simulink model "LKAS_AutoSave_DF_20220408_1006_SW62"  (R2018b)
settings: Solver=FixedStepDiscrete  StartTime=0.0  StopTime=10.0  FixedStep=0.01  RelTol=1e-3
undefined symbols (not defined in the file): LKA_CarWidth, LKA_SampleTime, LKA_StrRatio_C, LKA_Veh2CamL_C, LKA_Veh2CamW_C, LKA_WhlBaseL_C, LL_CompHdAg_C, LL_CompSWA_C, LL_CrvtPrvwT_C, LL_DesDvt_C, LL_DvtComp_C, LL_DvtPrvwT_C, LL_DvtSpdDet_vDvtSpdMin_C, LL_HandsOff_ExitTime, LL_HandsOff_TextTime, LL_HandsOff_WarnTime, LL_HdAgExT_C, LL_HdAgPrvwT_C, LL_LAccMax_C, LL_LAccRMax_C, LL_LDW_EarliestWarnLine_C, LL_LDW_LatestWarnLine_C, LL_LDWS_SUPPRESS_HEADING, LL_LFClb_TFC_FfCtlRatio_C, LL_LFClb_TFC_KdBalance_C, LL_LFClb_TFC_KdMaxSWA_C, LL_LFClb_TFC_KdV1_C, LL_LFClb_TFC_KdV2_C, LL_LFClb_TFC_KdVehSpdLwr_C, LL_LFClb_TFC_KdVehSpdUpr_C, LL_LFClb_TFC_Ki_C, LL_LFClb_TFC_KiMaxSWA_C, LL_LFClb_TFC_Kp_C, LL_LFClb_TFC_KpKlat_C, LL_LFClb_TFC_KpV1_C, LL_LFClb_TFC_KpV2_C, LL_LFClb_TFC_KpVehSpdLwr_C, LL_LFClb_TFC_KpVehSpdUpr_C, LL_LFClb_TFC_PrvwT_C, LL_LKA_EarliestWarnLine_C, LL_LKA_LatestWarnLine_C, LL_LKAExPrcs_ExitC0Dvt, LL_LKAExPrcs_ExitC0Swt, LL_LKAExPrcs_tiExitDelayTime3, LL_LKAExPrcs_tiExitTime1, LL_LKAExPrcs_tiExitTime2, LL_LKAExPrcs_tiExitTime3, LL_LKAS_OUT_OF_CONTROL_LAT_VEL, LL_LKAS_OUT_OF_CONTROL_TTLC, LL_LKASWASyn_M0, LL_LKASWASyn_M1, LL_LKASWASyn_M2, LL_LKASWASyn_M3D, LL_LKASWASyn_M3K_DT, LL_LKASWASyn_M3K_MSD, LL_LKASWASyn_M4K, LL_LKASWASyn_SWAaddMax, LL_LKASWASyn_T2, LL_LKASWASyn_tiTrqSwaRtTime, LL_LKASWASyn_tiTrqSwaTime ... (+47)
libraries: simulink x234, canmsglib x6, dspstat3 x3, simulink_extras x1
(part 5 of 16)

== system LKAS_AutoSave_DF_20220408_1006_SW62/LKAS/LL/Fault_Diagnostic/FuncFaultStatus_Unpack ==
  note: ob_ADIA_SpareDataCheck
  FuncFaultStatus : Inport
  Bus Creator : BusCreator  Inputs=16
  Extract Bits : simulink/Logic and Bit Operations/Extract Bits  bitsToExtract=Range of bits  numBits=8  bitIdxRange=0  outScalingMode=Treat bit field as an integer
      settings: SourceProductName=Simulink
  Extract Bits1 : simulink/Logic and Bit Operations/Extract Bits  bitsToExtract=Range of bits  numBits=8  bitIdxRange=1  outScalingMode=Treat bit field as an integer
      settings: SourceProductName=Simulink
  Extract Bits10 : simulink/Logic and Bit Operations/Extract Bits  bitsToExtract=Range of bits  numBits=8  bitIdxRange=10  outScalingMode=Treat bit field as an integer
      settings: SourceProductName=Simulink
  Extract Bits11 : simulink/Logic and Bit Operations/Extract Bits  bitsToExtract=Range of bits  numBits=8  bitIdxRange=11  outScalingMode=Treat bit field as an integer
      settings: SourceProductName=Simulink
  Extract Bits12 : simulink/Logic and Bit Operations/Extract Bits  bitsToExtract=Range of bits  numBits=8  bitIdxRange=12  outScalingMode=Treat bit field as an integer
      settings: SourceProductName=Simulink
  Extract Bits13 : simulink/Logic and Bit Operations/Extract Bits  bitsToExtract=Range of bits  numBits=8  bitIdxRange=13  outScalingMode=Treat bit field as an integer
      settings: SourceProductName=Simulink
  Extract Bits14 : simulink/Logic and Bit Operations/Extract Bits  bitsToExtract=Range of bits  numBits=8  bitIdxRange=14  outScalingMode=Treat bit field as an integer
      settings: SourceProductName=Simulink
  Extract Bits15 : simulink/Logic and Bit Operations/Extract Bits  bitsToExtract=Range of bits  numBits=8  bitIdxRange=15  outScalingMode=Treat bit field as an integer
      settings: SourceProductName=Simulink
  Extract Bits2 : simulink/Logic and Bit Operations/Extract Bits  bitsToExtract=Range of bits  numBits=8  bitIdxRange=2  outScalingMode=Treat bit field as an integer
      settings: SourceProductName=Simulink
  Extract Bits3 : simulink/Logic and Bit Operations/Extract Bits  bitsToExtract=Range of bits  numBits=8  bitIdxRange=3  outScalingMode=Treat bit field as an integer
      settings: SourceProductName=Simulink
  Extract Bits4 : simulink/Logic and Bit Operations/Extract Bits  bitsToExtract=Range of bits  numBits=8  bitIdxRange=4  outScalingMode=Treat bit field as an integer
      settings: SourceProductName=Simulink
  Extract Bits5 : simulink/Logic and Bit Operations/Extract Bits  bitsToExtract=Range of bits  numBits=8  bitIdxRange=5  outScalingMode=Treat bit field as an integer
      settings: SourceProductName=Simulink
  Extract Bits6 : simulink/Logic and Bit Operations/Extract Bits  bitsToExtract=Range of bits  numBits=8  bitIdxRange=6  outScalingMode=Treat bit field as an integer
      settings: SourceProductName=Simulink
  Extract Bits7 : simulink/Logic and Bit Operations/Extract Bits  bitsToExtract=Range of bits  numBits=8  bitIdxRange=7  outScalingMode=Treat bit field as an integer
      settings: SourceProductName=Simulink
  Extract Bits8 : simulink/Logic and Bit Operations/Extract Bits  bitsToExtract=Range of bits  numBits=8  bitIdxRange=8  outScalingMode=Treat bit field as an integer
      settings: SourceProductName=Simulink
  Extract Bits9 : simulink/Logic and Bit Operations/Extract Bits  bitsToExtract=Range of bits  numBits=8  bitIdxRange=9  outScalingMode=Treat bit field as an integer
      settings: SourceProductName=Simulink
  bsFuncFaultStatus : Outport
  wires:
  Extract Bits9/1 -> Bus Creator/10
  Extract Bits6/1 -> Bus Creator/7
  Extract Bits7/1 -> Bus Creator/8
  Extract Bits3/1 -> Bus Creator/4
  Extract Bits4/1 -> Bus Creator/5
  Extract Bits8/1 -> Bus Creator/9  "ob_ADIA_SpareDataCheck"
  Extract Bits15/1 -> Bus Creator/16  "ob_DTC_AEB_Safety_Violation"
  Bus Creator/1 -> bsFuncFaultStatus/1  "bsFuncFaultStatus"
  Extract Bits/1 -> Bus Creator/1
  Extract Bits12/1 -> Bus Creator/13  "ob_DTC_ACC_Mixed_Mode_Conflict"
  Extract Bits11/1 -> Bus Creator/12  "ob_DTC_ACC_Accel_Decel_Safety_Violation"
  Extract Bits10/1 -> Bus Creator/11
  Extract Bits14/1 -> Bus Creator/15  "ob_DTC_ACC_HoldConfirm_Safety_Violation"
  Extract Bits5/1 -> Bus Creator/6
  Extract Bits13/1 -> Bus Creator/14  "ob_DTC_ACC_Displacement_Safety_Violation"
  Extract Bits1/1 -> Bus Creator/2
  Extract Bits2/1 -> Bus Creator/3
  FuncFaultStatus/1 -> Extract Bits15/1, Extract Bits14/1, Extract Bits13/1, Extract Bits12/1, Extract Bits11/1, Extract Bits10/1, Extract Bits9/1, Extract Bits8/1, Extract Bits7/1, Extract Bits6/1, Extract Bits5/1, Extract Bits4/1, Extract Bits3/1, Extract Bits2/1, Extract Bits1/1, Extract Bits/1

== system LKAS_AutoSave_DF_20220408_1006_SW62/LKAS/LL/Human Machine Interface (HMI)/Subsystem ==
  LDW_State : Inport
  LKA_State : Inport  Port=2
  bsEPSInfo : Inport  Port=3
  LKA_SampleTime : Inport  Port=4
  LL_HandsOff_TextTime : Inport  Port=5
  LL_HandsOff_WarnTime : Inport  Port=6
  LL_RlsDet_tiTrqChkT_DISABLE : Inport  Port=7
  LL_RlsDet_tiTrqChkT_EPS_DISABLE : Inport  Port=8
  Abs : Abs
  Bus Selector2 : BusSelector  OutputSignals=EPS_LKA_State,EPS_SW_Trq
  Compare{1..2,4,7} (4 alike) : simulink/Logic and Bit Operations/Compare To Constant  relop===  const=3  OutDataTypeStr=boolean
  Compare3 : simulink/Logic and Bit Operations/Compare To Constant  relop===  const=1  OutDataTypeStr=boolean
  Compare5 : simulink/Logic and Bit Operations/Compare To Constant  relop===  const=4  OutDataTypeStr=boolean
  Compare6 : simulink/Logic and Bit Operations/Compare To Constant  relop===  const=5  OutDataTypeStr=boolean
  Compare8 : simulink/Logic and Bit Operations/Compare To Constant  relop===  const=4  OutDataTypeStr=boolean
  Compare9 : simulink/Logic and Bit Operations/Compare To Constant  relop===  const=5  OutDataTypeStr=boolean
  Logical Operator1 : Logic  Operator=OR  AllPortsSameDT=off  OutDataTypeStr=boolean
  Logical Operator2 : Logic  Inputs=3  AllPortsSameDT=off  OutDataTypeStr=boolean
  Logical Operator3 : Logic  Operator=OR  Inputs=6  AllPortsSameDT=off  OutDataTypeStr=boolean
  Relational Operator : RelationalOperator  Operator=<=  OutDataTypeStr=boolean  RndMeth=Nearest
  Sum Condition1 : Subsystem  TreatAsAtomicUnit=on
  Sum Condition2 : Subsystem  TreatAsAtomicUnit=on
  Switch : Switch  Criteria=u2 > Threshold
  HandsOff2_Warn : Outport
  HandsOff1_Text : Outport  Port=2
  wires:
  LKA_SampleTime/1 -> [LKA_SampleTime]
  Bus Selector2/2 -> Abs/1  "<EPS_SW_Trq>"
  LL_HandsOff_WarnTime/1 -> Sum Condition2/2(Sum)
  LL_HandsOff_TextTime/1 -> Sum Condition1/2(Sum)
  [LKA_SampleTime] -> Sum Condition2/1(SampleTime), Sum Condition1/1(SampleTime)
  Logical Operator1/1 -> Logical Operator2/2
  Compare3/1 -> Logical Operator1/2
  Compare2/1 -> Logical Operator1/1
  Compare7/1 -> Logical Operator3/6
  Compare8/1 -> Logical Operator3/5
  Compare9/1 -> Logical Operator3/4
  LKA_State/1 -> Compare7/1, Compare8/1, Compare9/1
  Abs/1 -> Relational Operator/1
  Compare6/1 -> Logical Operator3/1
  Compare5/1 -> Logical Operator3/2
  Compare4/1 -> Logical Operator3/3
  LDW_State/1 -> Compare5/1, Compare6/1, Compare4/1
  Sum Condition2/1(Out) -> HandsOff2_Warn/1
  Relational Operator/1 -> Logical Operator2/3
  LL_RlsDet_tiTrqChkT_DISABLE/1 -> Switch/3
  Logical Operator3/1 -> Logical Operator2/1
  Logical Operator2/1 -> Sum Condition1/Enable, Sum Condition2/Enable
  Compare1/1 -> Switch/2
  Switch/1 -> Relational Operator/2
  bsEPSInfo/1 -> Bus Selector2/1
  LL_RlsDet_tiTrqChkT_EPS_DISABLE/1 -> Switch/1
  Bus Selector2/1 -> Compare1/1, Compare2/1, Compare3/1  "<EPS_LKA_State>"
  Sum Condition1/1(Out) -> HandsOff1_Text/1

== system LKAS_AutoSave_DF_20220408_1006_SW62/LKAS/LL/LL Inputs Mapping/bsBCMInfo ==
  bsBCMInfoIn : Inport
  Bus Creator1 : BusCreator  Inputs=3
  Bus Selector1 : BusSelector  OutputSignals=BCM_Double_Light,BCM_Left_Light,BCM_Right_Light,BCM_LeftTurn_Switch,BCM_RightTurn_Switch
  Compare To Constant : simulink/Logic and Bit Operations/Compare To Constant  relop===  const=1  OutDataTypeStr=boolean
  Compare To Constant1 : simulink/Logic and Bit Operations/Compare To Constant  relop===  const=1  OutDataTypeStr=boolean
  Logical Operator : Logic  Operator=OR  AllPortsSameDT=off  OutDataTypeStr=boolean
  Logical Operator1 : Logic  Operator=OR  AllPortsSameDT=off  OutDataTypeStr=boolean
  bsBCMInfoOut : Outport
  wires:
  Logical Operator1/1 -> Bus Creator1/3  "BCM_Right_Light"
  Logical Operator/1 -> Bus Creator1/2  "BCM_Left_Light"
  Compare To Constant1/1 -> Logical Operator1/2
  Compare To Constant/1 -> Logical Operator/2
  Bus Selector1/5 -> Compare To Constant1/1  "<BCM_RightTurn_Switch>"
  Bus Selector1/4 -> Compare To Constant/1  "<BCM_LeftTurn_Switch>"
  bsBCMInfoIn/1 -> Bus Selector1/1
  Bus Selector1/1 -> Bus Creator1/1  "<BCM_Double_Light>"
  Bus Creator1/1 -> bsBCMInfoOut/1
  Bus Selector1/2 -> Logical Operator/1  "<BCM_Left_Light>"
  Bus Selector1/3 -> Logical Operator1/1  "<BCM_Right_Light>"

== system LKAS_AutoSave_DF_20220408_1006_SW62/LKAS/LL/LL Inputs Mapping/bsEPSInfo ==
  bsEPSInfoIn : Inport
  Bus Creator4 : BusCreator  Inputs=11
  Bus Selector1 : BusSelector  OutputSignals=EPS_LKA_State,EPS_SW_Trq,EPS_Trq_State,SAS_Clb_State,SAS_Trim_State,SWS_Failure_Status,EPS_TrqLim_State,EPS_LKA_Current,EPS_SWHold_State,EPS_Driver_Override,EPS_ESA_State
  bsEPSInfoOut : Outport
  wires:
  Bus Selector1/11 -> Bus Creator4/11  "<EPS_ESA_State>"
  Bus Selector1/10 -> Bus Creator4/10  "<EPS_Driver_Override>"
  Bus Selector1/6 -> Bus Creator4/6  "<SWS_Failure_Status>"
  bsEPSInfoIn/1 -> Bus Selector1/1
  Bus Selector1/2 -> Bus Creator4/2  "<EPS_SW_Trq>"
  Bus Selector1/1 -> Bus Creator4/1  "<EPS_LKA_State>"
  Bus Creator4/1 -> bsEPSInfoOut/1
  Bus Selector1/3 -> Bus Creator4/3  "<EPS_Trq_State>"
  Bus Selector1/4 -> Bus Creator4/4  "<SAS_Clb_State>"
  Bus Selector1/5 -> Bus Creator4/5  "<SAS_Trim_State>"
  Bus Selector1/7 -> Bus Creator4/7  "<EPS_TrqLim_State>"
  Bus Selector1/8 -> Bus Creator4/8  "<EPS_LKA_Current>"
  Bus Selector1/9 -> Bus Creator4/9  "<EPS_SWHold_State>"

== system LKAS_AutoSave_DF_20220408_1006_SW62/LKAS/LL/LL Inputs Mapping/bsLaneInfo ==
  bsLLClb : Inport
  bsLaneInfoIn : Inport  Port=2
  Bus Creator : BusCreator  Inputs=5
  Bus Selector1 : BusSelector  OutputSignals=bsFusL0Info,bsFusR0Info,bsFusL1Info,bsFusR1Info,bsFusLrgInfo,bsFusRrgInfo,Fusion_AdditionalInf
  LaneSelect : Subsystem
  "LanesReconstruct " : Subsystem
  bsLaneInfoOut : Outport
  wires:
  LaneSelect/6(bsRrgInfo) -> "LanesReconstruct "/7(bsRrgInfo)
  LaneSelect/5(bsLrgInfo) -> "LanesReconstruct "/6(bsLrgInfo)
  Bus Selector1/6 -> LaneSelect/6(bsFusRrgInfo)  "<bsFusRrgInfo>"
  Bus Selector1/5 -> LaneSelect/5(bsFusLrgInfo)  "<bsFusLrgInfo>"
  bsLLClb/1 -> "LanesReconstruct "/1(bsLLClb)
  bsLaneInfoIn/1 -> Bus Selector1/1
  Bus Selector1/7 -> Bus Creator/5  "<Fusion_AdditionalInf>"
  "LanesReconstruct "/1(bsL0InfoR) -> Bus Creator/1  "bsL0Info"
  "LanesReconstruct "/2(bsR0InfoR) -> Bus Creator/2  "bsR0Info"
  "LanesReconstruct "/3(bsL1InfoR) -> Bus Creator/3  "bsL1Info"
  "LanesReconstruct "/4(bsR1InfoR) -> Bus Creator/4  "bsR1Info"
  LaneSelect/1(bsL0Info) -> "LanesReconstruct "/2(bsL0Info)
  LaneSelect/2(bsR0Info) -> "LanesReconstruct "/3(bsR0Info)
  LaneSelect/3(bsL1Info) -> "LanesReconstruct "/4(bsL1Info)
  LaneSelect/4(bsR1Info) -> "LanesReconstruct "/5(bsR1Info)
  Bus Selector1/1 -> LaneSelect/1(bsFusL0Info)  "<bsFusL0Info>"
  Bus Selector1/2 -> LaneSelect/2(bsFusR0Info)  "<bsFusR0Info>"
  Bus Selector1/3 -> LaneSelect/3(bsFusL1Info)  "<bsFusL1Info>"
  Bus Selector1/4 -> LaneSelect/4(bsFusR1Info)  "<bsFusR1Info>"
  Bus Creator/1 -> bsLaneInfoOut/1

== system LKAS_AutoSave_DF_20220408_1006_SW62/LKAS/LL/LL Inputs Mapping/bsMP5Info ==
  note: ELK_Mode
      | 0: off
      | 1: LDW
      | 2: ~
      | 3: ELK
  note: LKA_Mode
      | 0: off
      | 1: LDW
      | 2: LKA
  note: LKA_Mode
      | 0: LDW
      | 1: LKA
      | 2: ~
  note: LkaFcnConf
      | 0: OFF
      | 1: LDW-声音
      | 2: LDW-振动
      | 3: LDW-声音+振动
      | 4: LKA-声音
      | 5: LKA-振动
      | 6: LKA-声音+振动
      | 7: LDW-声音-ICA
      | 8: LDW-振动-ICA
      | 9: LDW-声音+振动-ICA
      | 10: LKA-声音-ICA
      | 11: LKA-振动-ICA
      | 12: LKA-声音+振动-ICA
  note: LDW_Warn_Mode
      | 0: 声音
      | 1: 振动
      | 2: 声音+振动
  bsMP5InfoIn : Inport
  Bus Creator : BusCreator  Inputs=6
  Bus Selector1 : BusSelector  OutputSignals=LkaFcnConf,LKA_Main_Switch,LKA_Mode,LDW_Warn_Mode,APA_AutoPark_WorkSt,MP5_Work_State
  Cast To Boolean : DataTypeConversion  OutDataTypeStr=boolean
  MATLAB Function : MATLAB Function  TreatAsAtomicUnit=on
  bsMP5InfoOut : Outport
  wires:
  Cast To Boolean/1 -> MATLAB Function/2(LKA_Main_Switch_In)
  MATLAB Function/2(LKA_Switch) -> Bus Creator/2  "LKA_Switch"
  Bus Selector1/2 -> Cast To Boolean/1  "<LKA_Main_Switch>"
  Bus Selector1/1 -> MATLAB Function/1(LkaFcnConf)  "<LkaFcnConf>"
  MATLAB Function/1(LKA_Main_Switch) -> Bus Creator/1  "LKA_Main_Switch"
  MATLAB Function/4(LDW_Warn_Mode) -> Bus Creator/4  "LDW_Warn_Mode"
  MATLAB Function/3(LKA_Mode) -> Bus Creator/3  "LKA_Mode"
  Bus Selector1/4 -> MATLAB Function/4(LDW_Warn_Mode_In)  "<LDW_Warn_Mode>"
  Bus Selector1/3 -> MATLAB Function/3(LKA_Mode_In)  "<LKA_Mode>"
  Bus Creator/1 -> bsMP5InfoOut/1
  Bus Selector1/6 -> Bus Creator/6  "<MP5_Work_State>"
  Bus Selector1/5 -> Bus Creator/5  "<APA_AutoPark_WorkSt>"
  bsMP5InfoIn/1 -> Bus Selector1/1

== system LKAS_AutoSave_DF_20220408_1006_SW62/LKAS/LL/LL Inputs Mapping/bsPTState ==
  bsPTStateIn : Inport
  Bus Creator3 : BusCreator  Inputs=3
  Bus Selector1 : BusSelector  OutputSignals=AccPedal_Pos,TCU_ActualGear,TCU_Available
  Constant1 : Constant  Value=0  OutDataTypeStr=uint8
  Constant3 : Constant  Value=3  OutDataTypeStr=uint8
  Multiport Switch : MultiPortSwitch  DataPortOrder=Zero-based contiguous  Inputs=11  zeroidx=on
  bsPTStateOut : Outport
  wires:
  Bus Selector1/3 -> Bus Creator3/3  "<TCU_Available>"
  Constant1/1 -> Multiport Switch/2, Multiport Switch/7, Multiport Switch/8, Multiport Switch/12
  Bus Selector1/2 -> Multiport Switch/1  "<TCU_ActualGear>"
  Constant3/1 -> Multiport Switch/3, Multiport Switch/4, Multiport Switch/5, Multiport Switch/6, Multiport Switch/9, Multiport Switch/10, Multiport Switch/11
  Multiport Switch/1 -> Bus Creator3/2  "TCU_ActualGear"
  bsPTStateIn/1 -> Bus Selector1/1
  Bus Selector1/1 -> Bus Creator3/1  "<AccPedal_Pos>"
  Bus Creator3/1 -> bsPTStateOut/1

== system LKAS_AutoSave_DF_20220408_1006_SW62/LKAS/LL/LL Inputs Mapping/bsSWAInfo ==
  bsSWAInfoIn : Inport
  Bus Creator : BusCreator  Inputs=4
  Bus Selector1 : BusSelector  OutputSignals=EPS_SteeringAngle_Flag,EPS_SteeringAngle,SW_Angle,SW_Angle_Speed
  Gain : Gain
  bsSWAInfoOut : Outport
  wires:
  Bus Selector1/1 -> Bus Creator/1  "<EPS_SteeringAngle_Flag>"
  Bus Selector1/2 -> Gain/1, Bus Creator/2  "<EPS_SteeringAngle>"
  bsSWAInfoIn/1 -> Bus Selector1/1
  Gain/1 -> Bus Creator/3  "SW_Angle"
  Bus Selector1/4 -> Bus Creator/4  "<SW_Angle_Speed>"
  Bus Creator/1 -> bsSWAInfoOut/1

== system LKAS_AutoSave_DF_20220408_1006_SW62/LKAS/LL/LL Inputs Mapping/bsVehMovInfo ==
  bsVehMovInfoIn : Inport
  Bus Creator : BusCreator  Inputs=10
  Bus Selector2 : BusSelector  OutputSignals=ESC_LatAcc,ESC_LatAcc_Valid,ESC_YawRate,ESC_YawRate_Valid,ESC_UnYawRate,ESC_VehSpd,ESC_LonAcc,ESC_LonAcc_Valid,ESC_Brake_Press,ESC_VehSpd_Valid
  Saturation : Saturate  UpperLimit=inf  LowerLimit=0.1
  bsVehMovInfoOut : Outport
  wires:
  Saturation/1 -> Bus Creator/6  "ESC_VehSpd"
  bsVehMovInfoIn/1 -> Bus Selector2/1
  Bus Selector2/1 -> Bus Creator/1  "<ESC_LatAcc>"
  Bus Selector2/2 -> Bus Creator/2  "<ESC_LatAcc_Valid>"
  Bus Selector2/3 -> Bus Creator/3  "<ESC_YawRate>"
  Bus Selector2/4 -> Bus Creator/4  "<ESC_YawRate_Valid>"
  Bus Selector2/5 -> Bus Creator/5  "<ESC_UnYawRate>"
  Bus Selector2/6 -> Saturation/1  "<ESC_VehSpd>"
  Bus Selector2/7 -> Bus Creator/7  "<ESC_LonAcc>"
  Bus Selector2/8 -> Bus Creator/8  "<ESC_LonAcc_Valid>"
  Bus Selector2/9 -> Bus Creator/9  "<ESC_Brake_Press>"
  Bus Selector2/10 -> Bus Creator/10  "<ESC_VehSpd_Valid>"
  Bus Creator/1 -> bsVehMovInfoOut/1

== system LKAS_AutoSave_DF_20220408_1006_SW62/LKAS/LL/LLOn/LDW ==
  bsLKAInPInfo : Inport
  bsLLClb : Inport  Port=2
  Enable : EnablePort  StatesWhenEnabling=reset  ShowOutputPort=on
      settings: AttributesFormatString=states = %<StatesWhenEnabling>
  Bus Selector : BusSelector  OutputSignals=bsHdAgInfo.phiHdAg_Lft,bsHdAgInfo.phiHdAg_Rgt
  Bus Selector1 : BusSelector  OutputSignals=bsLDWClb.LL_LDWS_SUPPRESS_HEADING,bsConstantClb.LKA_SampleTime
  Cast : DataTypeConversion  OutDataTypeStr=uint8
  Heading Angle Detection (HdAgDet) : Subsystem  Description=|
      | Block Name: Heading Angle Detection
      | Ab.: HdAgDet
      | No.: 1.3.1.0
      | Rev: 0.0.1
      | Update Date: 19-3-26
  Logical Operator : Logic  Operator=NOT  AllPortsSameDT=off  OutDataTypeStr=boolean
  Product : Product  OutDataTypeStr=uint8
  LDW_Flag : Outport  OutputWhenDisabled=reset  InitialOutput=0
      settings: AttributesFormatString=%<OutputWhenDisabled> = %<InitialOutput>
  wires:
  Bus Selector1/1 -> Heading Angle Detection (HdAgDet)/4(LL_LDWS_SUPPRESS_HEADING)  "<LL_LDWS_SUPPRESS_HEADING>"
  bsLLClb/1 -> Bus Selector1/1
  Bus Selector/2 -> Heading Angle Detection (HdAgDet)/3(phiHdAg_Rgt)  "<phiHdAg_Rgt>"
  Bus Selector/1 -> Heading Angle Detection (HdAgDet)/2(phiHdAg_Lft)  "<phiHdAg_Lft>"
  Enable/1 -> Product/1, Heading Angle Detection (HdAgDet)/1(Enable)
  bsLKAInPInfo/1 -> Bus Selector/1
  Heading Angle Detection (HdAgDet)/1(stHdAgDetFlg) -> Logical Operator/1
  Product/1 -> LDW_Flag/1
  Bus Selector1/2 -> Heading Angle Detection (HdAgDet)/5(LKA_SampleTime)  "<LKA_SampleTime>"
  Cast/1 -> Product/2
  Logical Operator/1 -> Cast/1

== system LKAS_AutoSave_DF_20220408_1006_SW62/LKAS/LL/LLOn/LKA ==
  bsInInfo : Inport
  bsLKAInPInfo : Inport  Port=2
  bsLLClb : Inport  Port=3
  Enable : EnablePort  StatesWhenEnabling=reset  ShowOutputPort=on
      settings: AttributesFormatString=states = %<StatesWhenEnabling>
  Bus Selector : BusSelector  OutputSignals=bsConstantClb.LKA_SampleTime
  Cast To Single : DataTypeConversion  OutDataTypeStr=uint8
  Driver Torque Addition (DTA) : Subsystem
  LKA Exit Processing (LKAExPrcs) : Subsystem  Description=|
      | Block Name: LKA Exit Processing 
      | Ab.: LKAExPrcs
      | No.: 1.2.2.0
      | Rev: 0.0.1
      | Update Date: 19-5-13
  "LKA Motion Planning (LKAMP) " : Subsystem  Description=|
      | Block Name: LKA Motion Planning
      | Ab.: LKAMP
      | No.: 1.2.3.0
      | Rev: 0.0.1
      | Update Date: 19-5-13
  LKA SWA Limit (LKASWALim) : Subsystem  Description=|
      | Block Name: LKA SWA Synthesis
      | Ab.: LKASWASyn
      | No.: 1.2.6.0
      | Rev: 0.0.1
      | Update Date: 19-5-13
  LKA_Mon : Subsystem
  Lane Following (LF) : Subsystem  Description=|
      | Block Name: Lane Following
      | Ab.: LF
      | No.: 02
      | Rev: 00.00.01
      | Update Date: 19-3-28
  Plan To LaneFollowing (PTLF) : Subsystem
  LKA_ExitFlg : Outport  OutputWhenDisabled=reset  InitialOutput=0
      settings: AttributesFormatString=%<OutputWhenDisabled> = %<InitialOutput>
  LKA_phiSWACmd : Outport  Port=2  OutputWhenDisabled=reset  InitialOutput=0
      settings: AttributesFormatString=%<OutputWhenDisabled> = %<InitialOutput>
  LKA_M : Outport  Port=3  OutputWhenDisabled=reset  InitialOutput=0
      settings: AttributesFormatString=%<OutputWhenDisabled> = %<InitialOutput>
  LKAMon : Outport  Port=4  OutputWhenDisabled=reset  InitialOutput=0
      settings: AttributesFormatString=%<OutputWhenDisabled> = %<InitialOutput>
  tag scope: ActFlg=global, Ff=global, LKA_ExitFlg_Mon=global, LKA_SampleTime=global, PT1=global
  wires:
  [LKA_Exit3Flg] -> Driver Torque Addition (DTA)/3(DTA_Exit3Flg)
  LKA Exit Processing (LKAExPrcs)/3(LKAExPrcs_stExit3Flg) -> [LKA_Exit3Flg]
  [Ff] -> "LKA Motion Planning (LKAMP) "/2(LKAMP_Ff)
  Bus Selector/1 -> [LKA_SampleTime]  "<LKA_SampleTime>"
  [LKA_bsLLClb] -> "LKA Motion Planning (LKAMP) "/5(LKAMP_bsLLClb)
  LKA_Mon/1(LKAMon) -> LKAMon/1
  "LKA Motion Planning (LKAMP) "/2(LKAMP_tiT1) -> [PT1]  "PlanT1"
  "LKA Motion Planning (LKAMP) "/1(LKAMP_phiSWACmd) -> [Plan]  "PlanSWACmd"
  Lane Following (LF)/4(LF_phiDiffSWACmd) -> [D]
  Lane Following (LF)/2(LF_phiPropSWACmd) -> [P]
  Lane Following (LF)/1(LF_phiFfLFSWACmd) -> [Ff]
  Lane Following (LF)/3(LF_phiIntegSWACmd) -> [I]
  Driver Torque Addition (DTA)/2(DTA_M) -> LKA_M/1
  [LKAInPInfo] -> Lane Following (LF)/2(LF_bsLKAInPInfo)
  [Ff] -> LKA SWA Limit (LKASWALim)/2(LKASWALim_Ff)
  [LKA_bsInInfoSyn] -> Lane Following (LF)/1(LF_bsInInfoSyn)
  [LKA_bsInInfoSyn] -> Driver Torque Addition (DTA)/1(DTA_bsInInfoSyn)
  [LKA_bsInInfoSyn] -> "LKA Motion Planning (LKAMP) "/1(LKAMP_bsInInfoSyn)
  bsInInfo/1 -> [LKA_bsInInfoSyn]
  [LKA_bsLLClb] -> LKA SWA Limit (LKASWALim)/4(LKASWALim_bsLKAClb)
  [LKA_bsLLClb] -> Lane Following (LF)/3(LF_bsLFClb)
  [LKA_bsLLClb] -> Driver Torque Addition (DTA)/2(DTA_bsLFClb)
  [LKA_bsLLClb] -> LKA Exit Processing (LKAExPrcs)/2(LKAExPrcs_bsLKAClb)
  [LKAInPInfo] -> LKA SWA Limit (LKASWALim)/3(LKASWALim_bsLKAInPInfo)
  bsLLClb/1 -> [LKA_bsLLClb], Bus Selector/1
  [LKAInPInfo] -> Plan To LaneFollowing (PTLF)/1(InP)
  [LKAInPInfo] -> LKA Exit Processing (LKAExPrcs)/1(LKAExPrcs_bsLKAInPInfo)
  [LKAInPInfo] -> "LKA Motion Planning (LKAMP) "/4(LKAMP_bsLKAInPInfo)
  bsLKAInPInfo/1 -> [LKAInPInfo]
  [ActFlg] -> "LKA Motion Planning (LKAMP) "/3(LKAMP_stLKAActvFlg)
  [PT1] -> LKA Exit Processing (LKAExPrcs)/3(LKAExPrcs_PlanT1)
  [PT1] -> Plan To LaneFollowing (PTLF)/3(T1)
  [Plan] -> Plan To LaneFollowing (PTLF)/2(Plan)
  [DT] -> Plan To LaneFollowing (PTLF)/4(DrvTrq)
  Driver Torque Addition (DTA)/1(DTA_phiDTASWACmd) -> [DT]  "DT"
  [D] -> Plan To LaneFollowing (PTLF)/8(D)
  [I] -> Plan To LaneFollowing (PTLF)/7(I)
  [P] -> Plan To LaneFollowing (PTLF)/6(P)
  [Ff] -> Plan To LaneFollowing (PTLF)/5(Ff)
  LKA Exit Processing (LKAExPrcs)/1(LKAExPrcs_stExFlg) -> [LKA_ExitFlg_Mon], LKA_ExitFlg/1
  LKA SWA Limit (LKASWALim)/1(LKASWALim_phiSWACmd) -> LKA_phiSWACmd/1  "phiSWACmd"
  Enable/1 -> Cast To Single/1
  Plan To LaneFollowing (PTLF)/1(SWACmd) -> LKA SWA Limit (LKASWALim)/1(LKASWALim_phiTFCSWACmd)  "PTLFSWACmd"
  Cast To Single/1 -> [ActFlg]  "ActFlg"

== system LKAS_AutoSave_DF_20220408_1006_SW62/LKAS/LL/LLOn/LKA Input Processing (LKAInP) ==
  bsInInfo : Inport
  bsLLClb : Inport  Port=2
  ActFlg : Inport  Port=3
  Bus Creator2 : BusCreator  Inputs=10
  Curvature Calculation (Crvt) : Subsystem
  Delay : Delay  DelayLength=1
  Deviation Calculation (Dvt) : Subsystem
  Heading Angle Calculation (HdAg) : Subsystem
  Lane Width Calculation (LW) : Subsystem
  Previewed Curvature Calculation (PrCrvt) : Subsystem
  Previewed Deviation Calculation (PrDvt) : Subsystem
  Previewed Heading Angle Calculation (PrHdAg) : Subsystem
  Steering Wheel Position Calculation (SWAPosCal) : Subsystem
  TTLC Calculation (TTLCCalc) : Subsystem  Description=|
      | Block Name: TTLC Calculation
      | Ab.: TTLCCalc
      | No.: 1.1.1.1
      | Rev: 0.0.1
      | Update Date: 19-3-26
  Under The Limit (UndrLim) : Subsystem
  bsLKAInPInfo : Outport
  wires:
  [bsTTLCInfo] -> Previewed Heading Angle Calculation (PrHdAg)/3(PrHdAg_bsTTLCInfo)  "bsTTLCInfo"
  TTLC Calculation (TTLCCalc)/1(TTLCCalc_bsTTLCInfo) -> [bsTTLCInfo]  "bsTTLCInfo"
  Previewed Deviation Calculation (PrDvt)/1(PrvwDvt_bsPrvwDvtInfo) -> [bsPrDvtInfo]  "bsPrDvtInfo"
  Previewed Heading Angle Calculation (PrHdAg)/1(PrHdAg_bsPrHdAgInfo) -> [bsPrHdAgInfo]  "bsPrHdAgInfo"
  [bsPrCrvtInfo] -> TTLC Calculation (TTLCCalc)/4(TTLCCalc_bsPrCrvtInfo)  "bsPrCrvtInfo"
  Previewed Curvature Calculation (PrCrvt)/1(PrvwCrvt_bsPrvwCrvtInfo) -> [bsPrCrvtInfo]  "bsPrCrvtInfo"
  [bsDvtInfo] -> TTLC Calculation (TTLCCalc)/1(TTLCCalc_bsDvtInfo)  "bsDvtInfo"
  Deviation Calculation (Dvt)/1(Dvt_bsDvtInfo) -> [bsDvtInfo]  "bsDvtInfo"
  [bsHdAgInfo] -> TTLC Calculation (TTLCCalc)/5(TTLCCalc_bsHdAgInfo)  "bsHdAgInfo"
  Heading Angle Calculation (HdAg)/1(HdAg_bsHdAgInfo) -> [bsHdAgInfo]  "bsHdAgInfo"
  Curvature Calculation (Crvt)/1(Crvt_bsCrvtInfo) -> [bsCrvtInfo]  "bsCrvtInfo"
  Under The Limit (UndrLim)/1(UndrLim_bsUndrLimInfo) -> [bsUndrLimInfo]  "bsUndrLimInfo"
  Steering Wheel Position Calculation (SWAPosCal)/1(SWAPosCal) -> [phiSWAPos]  "phiSWAPos"
  Lane Width Calculation (LW)/1(LW_LaneWidth) -> [LaneWidth]  "LaneWidth"
  Delay/1 -> Previewed Curvature Calculation (PrCrvt)/3(PrvwCrvt_stLKAActvFlg)
  ActFlg/1 -> Delay/1
  Bus Creator2/1 -> bsLKAInPInfo/1
  [bsPrCrvtInfo] -> Bus Creator2/7  "bsPrCrvtInfo"
  [bsPrDvtInfo] -> Bus Creator2/9  "bsPrDvtInfo"
  [bsCrvtInfo] -> Bus Creator2/4  "bsCrvtInfo"
  [bsDvtInfo] -> Bus Creator2/6  "bsDvtInfo"
  [bsUndrLimInfo] -> Bus Creator2/3  "bsUndrLimInfo"
  [phiSWAPos] -> Bus Creator2/2  "phiSWAPos"
  [LaneWidth] -> Bus Creator2/1  "LaneWidth"
  [bsTTLCInfo] -> Bus Creator2/10  "bsTTLCInfo"
  [bsPrHdAgInfo] -> Bus Creator2/8  "bsPrHdAgInfo"
  bsLLClb/1 -> TTLC Calculation (TTLCCalc)/2(TTLCCalc_bsLLClb), Previewed Curvature Calculation (PrCrvt)/2(PrvwCrvt_tiCrvtPrvwT_C), Steering Wheel Position Calculation (SWAPosCal)/2(SWAPosCal_bsLLClb), Under The Limit (UndrLim)/2(UndrLim_bsLLClb), Deviation Calculation (Dvt)/2(Dvt_bsLLClb), Previewed Heading Angle Calculation (PrHdAg)/2(PrHdAg_bsLLClb), Previewed Deviation Calculation (PrDvt)/1(PrdcDvt_bsLLClb)
  [bsHdAgInfo] -> Bus Creator2/5  "bsHdAgInfo"
  bsInInfo/1 -> Steering Wheel Position Calculation (SWAPosCal)/1(SWAPosCal_bsInInfoSyn), Lane Width Calculation (LW)/1(LW_bsInInfoSyn), Under The Limit (UndrLim)/1(UndrLim_bsInInfoSyn), Curvature Calculation (Crvt)/1(PrvwCrvt_bsInInfoSyn), Heading Angle Calculation (HdAg)/1(HdAg_bsInInfoSyn), Deviation Calculation (Dvt)/1(Dvt_bsInInfoSyn), Previewed Curvature Calculation (PrCrvt)/1(PrvwCrvt_bsInInfoSyn), Previewed Deviation Calculation (PrDvt)/2(PrvwDvt_bsInInfoSyn), TTLC Calculation (TTLCCalc)/3(TTLCCalc_bsInfo), Previewed Heading Angle Calculation (PrHdAg)/1(PrHdAg_bsInInfoSyn)

== system LKAS_AutoSave_DF_20220408_1006_SW62/LKAS/LL/LLOn/LL State Determination (LLStateDet) ==
  bsInInfo : Inport
  bsLKAInPInfo : Inport  Port=2
  bsLLClb : Inport  Port=3
  ExitFlg : Inport  Port=4
  bsSignalFault : Inport  Port=5
  Bus Creator : BusCreator  Inputs=3
  Delay : Delay  DelayLength=1
  Delay1 : Delay  DelayLength=1
  LDW_State_Machine : Stateflow chart  Description=|  TreatAsAtomicUnit=on
      | Block Name: LDW State Machine
      | Ab.: LDWSM
      | No.: 1.1.2.0
      | Rev: 0.0.1
      | Update Date: 19-3-26
      settings: RTWSystemCode=Nonreusable function
  LKA_State_Machine : Stateflow chart  Description=|  TreatAsAtomicUnit=on
      | Block Name: LKA State Machine
      | Ab.: LKASM
      | No.: 1.1.3.0
      | Rev: 0.0.1
      | Update Date: 19-3-26
      settings: RTWSystemCode=Nonreusable function
  LL State Machine Conditions (LLSMCon) : Subsystem
  bsLLState : Outport
  stLDWActvFlg : Outport  Port=2
  stLKAActvFlg : Outport  Port=3
  Disable_Reason : Outport  Port=4
  Fault_Reason : Outport  Port=5
  tag scope: LDW_State_Mon=global, LKA_State_Mon=global
  wires:
  [LKA_Mode] -> Bus Creator/2
  [LKA_Mode] -> LKA_State_Machine/1(LKA_Mode)
  [LKA_Mode] -> LDW_State_Machine/1(LKA_Mode)
  LL State Machine Conditions (LLSMCon)/1(LKA_Mode) -> [LKA_Mode]  "LKA_Mode"
  LL State Machine Conditions (LLSMCon)/13(Fault_Reason) -> Fault_Reason/1
  LL State Machine Conditions (LLSMCon)/12(Disable_Reason) -> Disable_Reason/1
  bsSignalFault/1 -> LL State Machine Conditions (LLSMCon)/6(bsSignalFault)
  Delay/1 -> LL State Machine Conditions (LLSMCon)/5(ExitFlg)
  bsLLClb/1 -> LL State Machine Conditions (LLSMCon)/3(bsLLClb)
  ExitFlg/1 -> Delay/1
  bsLKAInPInfo/1 -> LL State Machine Conditions (LLSMCon)/2(bsLKAInPInfo)
  bsInInfo/1 -> LL State Machine Conditions (LLSMCon)/1(bsInInfo)
  LL State Machine Conditions (LLSMCon)/11(LKA_Fault) -> LKA_State_Machine/6(LKA_Fault)
  LL State Machine Conditions (LLSMCon)/10(stLKADeactvCSyn) -> LKA_State_Machine/5(stLKADeactvCSyn)
  LL State Machine Conditions (LLSMCon)/9(stLKAActvCSyn) -> LKA_State_Machine/4(stLKAActvCSyn)
  LL State Machine Conditions (LLSMCon)/8(stLKADisblCSyn) -> LKA_State_Machine/3(stLKADisblCSyn)
  LL State Machine Conditions (LLSMCon)/7(stLKAEnaCSyn) -> LKA_State_Machine/2(stLKAEnaCSyn)
  LL State Machine Conditions (LLSMCon)/6(LDW_Fault) -> LDW_State_Machine/6(LDW_Fault)
  LDW_State_Machine/2(stLDWState) -> Bus Creator/1, [LDW_State_Mon]  "LDW_State"
  LKA_State_Machine/2(stLKAState) -> [LKA_State_Mon], Bus Creator/3  "LKA_State"
  Bus Creator/1 -> Delay1/1, bsLLState/1  "bsLLState"
  Delay1/1 -> LL State Machine Conditions (LLSMCon)/4(bsLLState)
  LKA_State_Machine/1(stLKAActvFlg) -> stLKAActvFlg/1
  LDW_State_Machine/1(stLDWActvFlg) -> stLDWActvFlg/1
  LL State Machine Conditions (LLSMCon)/5(stLDWDeactvCSyn) -> LDW_State_Machine/5(stLDWDeactvCSyn)  "stLDWDeactvCSyn"
  LL State Machine Conditions (LLSMCon)/4(stLDWActvCSyn) -> LDW_State_Machine/4(stLDWActvCSyn)
  LL State Machine Conditions (LLSMCon)/3(stLDWDisblCSyn) -> LDW_State_Machine/3(stLDWDisblCSyn)
  LL State Machine Conditions (LLSMCon)/2(stLDWEnaCSyn) -> LDW_State_Machine/2(stLDWEnaCSyn)

== system LKAS_AutoSave_DF_20220408_1006_SW62/LKAS/LL/LLOn/LL_Mon ==
  Disable_Reason : Inport
  Fault_Reason : Inport  Port=2
  LKAMon : Inport  Port=3
  Bus : BusCreator  Inputs=5
  BusInP : BusCreator  Inputs=2
  BusState : BusCreator  Inputs=2
  LLMon : Outport
  wires:
  Fault_Reason/1 -> Bus/5  "Fault_Reason"
  Disable_Reason/1 -> Bus/4  "Disable_Reason"
  BusState/1 -> [StateMon]  "StateMon"
  BusInP/1 -> [InPMon]  "InPMon"
  [LKA_State_Mon] -> BusState/2  "LKA_State_Mon"
  [LDW_State_Mon] -> BusState/1  "LDW_State_Mon"
  [RGTTTLC_Mon] -> BusInP/2  "RGTTTLC_Mon"
  [LFTTTLC_Mon] -> BusInP/1  "LFTTTLC_Mon"
  Bus/1 -> LLMon/1  "LLMon"
  LKAMon/1 -> Bus/3
  [StateMon] -> Bus/2
  [InPMon] -> Bus/1

== system LKAS_AutoSave_DF_20220408_1006_SW62/LKAS/LL/LLOut/Angle2Trq ==
  LKA_Torque_Req : Inport
  Target_Angle : Inport  Port=2
  Stearing_Angle : Inport  Port=3
  Constant : Constant  Value=5  OutDataTypeStr=single
  Constant1 : Constant  Value=-5  OutDataTypeStr=single
  Constant3 : Constant  Value=5  OutDataTypeStr=single
  Constant4 : Constant  Value=-5  OutDataTypeStr=single
  Rate Limiter Dynamic : Subsystem
  Saturation Dynamic : Subsystem
  Subsystem : Subsystem
  torque : Outport  OutputWhenDisabled=reset  InitialOutput=0
  wires:
  LKA_Torque_Req/1 -> Subsystem/Enable  "LKA_Torque_Req"
  Subsystem/1(in_trq) -> Rate Limiter Dynamic/2(u)  "in_trq"
  Stearing_Angle/1 -> Subsystem/2(Stearing_Angle)  "Stearing_Angle"
  Target_Angle/1 -> Subsystem/1(Target_Angle)  "Target_Angle"
  Constant/1 -> Rate Limiter Dynamic/1(up)
  Constant1/1 -> Rate Limiter Dynamic/3(lo)
  Rate Limiter Dynamic/1(Y) -> Saturation Dynamic/2(u)  "RL_trq"
  Constant3/1 -> Saturation Dynamic/1(up)
  Constant4/1 -> Saturation Dynamic/3(lo)
  Saturation Dynamic/1(y) -> torque/1  "Saturation_trq"

== system LKAS_AutoSave_DF_20220408_1006_SW62/LKAS/LLClb/LLSMConClb/ICv to v10 ==
  In1 : Inport
  Add : Sum  Inputs=+-
  Constant : Constant  Value=2.5  OutDataTypeStr=single
  Gain : Gain  Gain=1/1.02
  Out1 : Outport
  wires:
  Gain/1 -> Out1/1
  Constant/1 -> Add/2
  Add/1 -> Gain/1
  In1/1 -> Add/1

== system LKAS_AutoSave_DF_20220408_1006_SW62/LKAS/LLClb/LLSMConClb/ICv to v11 ==
  In1 : Inport
  Add : Sum  Inputs=+-
  Constant : Constant  Value=2.5  OutDataTypeStr=single
  Gain : Gain  Gain=1/1.02
  Out1 : Outport
  wires:
  In1/1 -> Add/1
  Add/1 -> Gain/1
  Constant/1 -> Add/2
  Gain/1 -> Out1/1

== system LKAS_AutoSave_DF_20220408_1006_SW62/LKAS/LLClb/LLSMConClb/ICv to v6 ==
  In1 : Inport
  Add : Sum  Inputs=+-
  Constant : Constant  Value=2.5  OutDataTypeStr=single
  Gain : Gain  Gain=1/1.02
  Out1 : Outport
  wires:
  Gain/1 -> Out1/1
  Constant/1 -> Add/2
  Add/1 -> Gain/1
  In1/1 -> Add/1

== system LKAS_AutoSave_DF_20220408_1006_SW62/LKAS/LLClb/LLSMConClb/ICv to v7 ==
  In1 : Inport
  Add : Sum  Inputs=+-
  Constant : Constant  Value=2.5  OutDataTypeStr=single
  Gain : Gain  Gain=1/1.02
  Out1 : Outport
  wires:
  In1/1 -> Add/1
  Add/1 -> Gain/1
  Constant/1 -> Add/2
  Gain/1 -> Out1/1

== system LKAS_AutoSave_DF_20220408_1006_SW62/LKAS/LLClb/LLSMConClb/ICv to v8 ==
  In1 : Inport
  Add : Sum  Inputs=+-
  Constant : Constant  Value=2.5  OutDataTypeStr=single
  Gain : Gain  Gain=1/1.02
  Out1 : Outport
  wires:
  Gain/1 -> Out1/1
  Constant/1 -> Add/2
  Add/1 -> Gain/1
  In1/1 -> Add/1

== system LKAS_AutoSave_DF_20220408_1006_SW62/LKAS/LLClb/LLSMConClb/ICv to v9 ==
  In1 : Inport
  Add : Sum  Inputs=+-
  Constant : Constant  Value=2.5  OutDataTypeStr=single
  Gain : Gain  Gain=1/1.02
  Out1 : Outport
  wires:
  In1/1 -> Add/1
  Add/1 -> Gain/1
  Constant/1 -> Add/2
  Gain/1 -> Out1/1

== system LKAS_AutoSave_DF_20220408_1006_SW62/LKAS/LL/Human Machine Interface (HMI)/Subsystem/Sum Condition1 ==
  SampleTime : Inport
  Sum : Inport  Port=2
  state = reset : EnablePort  StatesWhenEnabling=reset
  Add1 : Sum  OutDataTypeStr=single
  Memory : Memory  InheritSampleTime=on
  Relational Operator : RelationalOperator  OutDataTypeStr=boolean  RndMeth=Nearest
  Saturation : Saturate  UpperLimit=60  LowerLimit=0
      settings: AttributesFormatString="Min = %<LowerLimit>  Max = %<UpperLimit>"
  Out : Outport  OutputWhenDisabled=reset  InitialOutput=0
      settings: AttributesFormatString=%<OutputWhenDisabled> = %<InitialOutput>
  wires:
  SampleTime/1 -> Add1/1
  Saturation/1 -> Relational Operator/1, Memory/1
  Relational Operator/1 -> Out/1
  Sum/1 -> Relational Operator/2
  Add1/1 -> Saturation/1
  Memory/1 -> Add1/2

== system LKAS_AutoSave_DF_20220408_1006_SW62/LKAS/LL/Human Machine Interface (HMI)/Subsystem/Sum Condition2 ==
  SampleTime : Inport
  Sum : Inport  Port=2
  state = reset : EnablePort  StatesWhenEnabling=reset
  Add1 : Sum  OutDataTypeStr=single
  Memory : Memory  InheritSampleTime=on
  Relational Operator : RelationalOperator  OutDataTypeStr=boolean  RndMeth=Nearest
  Saturation : Saturate  UpperLimit=60  LowerLimit=0
      settings: AttributesFormatString="Min = %<LowerLimit>  Max = %<UpperLimit>"
  Out : Outport  OutputWhenDisabled=reset  InitialOutput=0
      settings: AttributesFormatString=%<OutputWhenDisabled> = %<InitialOutput>
  wires:
  Memory/1 -> Add1/2
  Add1/1 -> Saturation/1
  Sum/1 -> Relational Operator/2
  Relational Operator/1 -> Out/1
  Saturation/1 -> Memory/1, Relational Operator/1
  SampleTime/1 -> Add1/1

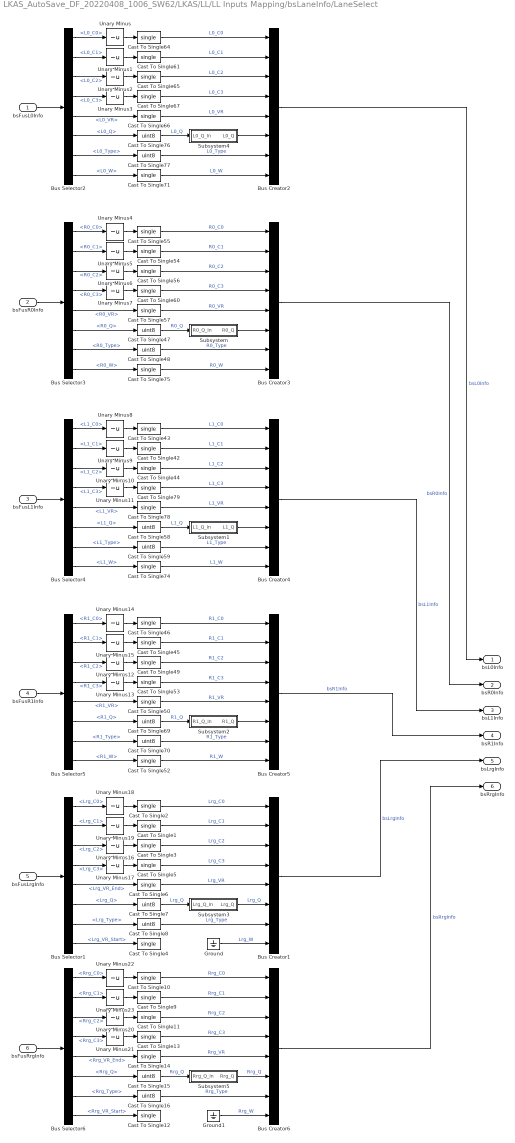
== system LKAS_AutoSave_DF_20220408_1006_SW62/LKAS/LL/LL Inputs Mapping/bsLaneInfo/LaneSelect ==
  bsFusL0Info : Inport
  bsFusR0Info : Inport  Port=2
  bsFusL1Info : Inport  Port=3
  bsFusR1Info : Inport  Port=4
  bsFusLrgInfo : Inport  Port=5
  bsFusRrgInfo : Inport  Port=6
  Bus Creator{1..6} (6 alike) : BusCreator  Inputs=8
  Bus Selector1 : BusSelector  OutputSignals=Lrg_C0,Lrg_C1,Lrg_C2,Lrg_C3,Lrg_VR_End,Lrg_Q,Lrg_Type,Lrg_VR_Start
  Bus Selector2 : BusSelector  OutputSignals=L0_C0,L0_C1,L0_C2,L0_C3,L0_VR,L0_Q,L0_Type,L0_W
  Bus Selector3 : BusSelector  OutputSignals=R0_C0,R0_C1,R0_C2,R0_C3,R0_VR,R0_Q,R0_Type,R0_W
  Bus Selector4 : BusSelector  OutputSignals=L1_C0,L1_C1,L1_C2,L1_C3,L1_VR,L1_Q,L1_Type,L1_W
  Bus Selector5 : BusSelector  OutputSignals=R1_C0,R1_C1,R1_C2,R1_C3,R1_VR,R1_Q,R1_Type,R1_W
  Bus Selector6 : BusSelector  OutputSignals=Rrg_C0,Rrg_C1,Rrg_C2,Rrg_C3,Rrg_VR_End,Rrg_Q,Rrg_Type,Rrg_VR_Start
  Cast To Single{1..6,9..14,42..46,49..50,52..57,60..61,64..67,71,74..75,78..79} (36 alike) : DataTypeConversion  OutDataTypeStr=single
  Cast To Single{7..8,15..16,47..48,58..59,69..70,76..77} (12 alike) : DataTypeConversion  OutDataTypeStr=uint8
  Ground : Ground
  Ground1 : Ground
  Subsystem : Subsystem
  Subsystem1 : Subsystem
  Subsystem2 : Subsystem
  Subsystem3 : Subsystem
  Subsystem4 : Subsystem
  Subsystem5 : Subsystem
  Unary Minus{,1..23} (24 alike) : UnaryMinus
  bsL0Info : Outport
  bsR0Info : Outport  Port=2
  bsL1Info : Outport  Port=3
  bsR1Info : Outport  Port=4
  bsLrgInfo : Outport  Port=5
  bsRrgInfo : Outport  Port=6
  wires:
  Subsystem5/1(Rrg_Q) -> Bus Creator6/6  "Rrg_Q"
  Subsystem3/1(Lrg_Q) -> Bus Creator1/6  "Lrg_Q"
  Unary Minus23/1 -> Cast To Single9/1
  Unary Minus22/1 -> Cast To Single10/1
  Unary Minus21/1 -> Cast To Single13/1
  Unary Minus20/1 -> Cast To Single11/1
  Unary Minus17/1 -> Cast To Single5/1
  Unary Minus19/1 -> Cast To Single1/1
  Unary Minus18/1 -> Cast To Single2/1
  Unary Minus16/1 -> Cast To Single3/1
  Bus Creator6/1 -> bsRrgInfo/1  "bsRrgInfo"
  Bus Creator1/1 -> bsLrgInfo/1  "bsLrgInfo"
  Ground1/1 -> Bus Creator6/8  "Rrg_W"
  Cast To Single16/1 -> Bus Creator6/7  "Rrg_Type"
  Cast To Single15/1 -> Subsystem5/1(Rrg_Q_In)  "Rrg_Q"
  Cast To Single14/1 -> Bus Creator6/5  "Rrg_VR"
  Cast To Single13/1 -> Bus Creator6/4  "Rrg_C3"
  Cast To Single11/1 -> Bus Creator6/3  "Rrg_C2"
  Cast To Single9/1 -> Bus Creator6/2  "Rrg_C1"
  Cast To Single10/1 -> Bus Creator6/1  "Rrg_C0"
  Bus Selector6/7 -> Cast To Single16/1  "<Rrg_Type>"
  Bus Selector6/6 -> Cast To Single15/1  "<Rrg_Q>"
  Bus Selector6/5 -> Cast To Single14/1  "<Rrg_VR_End>"
  Bus Selector6/8 -> Cast To Single12/1  "<Rrg_VR_Start>"
  Bus Selector6/4 -> Unary Minus21/1  "<Rrg_C3>"
  Bus Selector6/3 -> Unary Minus20/1  "<Rrg_C2>"
  Bus Selector6/2 -> Unary Minus23/1  "<Rrg_C1>"
  Bus Selector6/1 -> Unary Minus22/1  "<Rrg_C0>"
  Ground/1 -> Bus Creator1/8  "Lrg_W"
  Cast To Single8/1 -> Bus Creator1/7  "Lrg_Type"
  Cast To Single7/1 -> Subsystem3/1(Lrg_Q_In)  "Lrg_Q"
  Cast To Single5/1 -> Bus Creator1/4  "Lrg_C3"
  Cast To Single6/1 -> Bus Creator1/5  "Lrg_VR"
  Cast To Single2/1 -> Bus Creator1/1  "Lrg_C0"
  Cast To Single3/1 -> Bus Creator1/3  "Lrg_C2"
  Cast To Single1/1 -> Bus Creator1/2  "Lrg_C1"
  Bus Selector1/7 -> Cast To Single8/1  "<Lrg_Type>"
  Bus Selector1/6 -> Cast To Single7/1  "<Lrg_Q>"
  Bus Selector1/5 -> Cast To Single6/1  "<Lrg_VR_End>"
  Bus Selector1/8 -> Cast To Single4/1  "<Lrg_VR_Start>"
  Bus Selector1/4 -> Unary Minus17/1  "<Lrg_C3>"
  Bus Selector1/3 -> Unary Minus16/1  "<Lrg_C2>"
  Bus Selector1/2 -> Unary Minus19/1  "<Lrg_C1>"
  Bus Selector1/1 -> Unary Minus18/1  "<Lrg_C0>"
  bsFusRrgInfo/1 -> Bus Selector6/1
  bsFusLrgInfo/1 -> Bus Selector1/1
  Subsystem2/1(R1_Q) -> Bus Creator5/6
  Subsystem1/1(L1_Q) -> Bus Creator4/6
  Unary Minus15/1 -> Cast To Single45/1
  Unary Minus14/1 -> Cast To Single46/1
  Unary Minus13/1 -> Cast To Single53/1
  Unary Minus12/1 -> Cast To Single49/1
  Unary Minus10/1 -> Cast To Single44/1
  Unary Minus11/1 -> Cast To Single79/1
  Unary Minus9/1 -> Cast To Single42/1
  Unary Minus8/1 -> Cast To Single43/1
  Unary Minus5/1 -> Cast To Single54/1
  Unary Minus4/1 -> Cast To Single55/1
  Unary Minus6/1 -> Cast To Single56/1
  Unary Minus7/1 -> Cast To Single60/1
  Unary Minus3/1 -> Cast To Single67/1
  Unary Minus2/1 -> Cast To Single65/1
  Unary Minus1/1 -> Cast To Single61/1
  Unary Minus/1 -> Cast To Single64/1
  Cast To Single71/1 -> Bus Creator2/8  "L0_W"
  Cast To Single70/1 -> Bus Creator5/7  "R1_Type"
  Cast To Single69/1 -> Subsystem2/1(R1_Q_In)  "R1_Q"
  Cast To Single53/1 -> Bus Creator5/4  "R1_C3"
  Cast To Single52/1 -> Bus Creator5/8  "R1_W"
  Cast To Single50/1 -> Bus Creator5/5  "R1_VR"
  Cast To Single49/1 -> Bus Creator5/3  "R1_C2"
  Cast To Single46/1 -> Bus Creator5/1  "R1_C0"
  Cast To Single45/1 -> Bus Creator5/2  "R1_C1"
  Cast To Single74/1 -> Bus Creator4/8  "L1_W"
  Cast To Single79/1 -> Bus Creator4/4  "L1_C3"
  Cast To Single78/1 -> Bus Creator4/5  "L1_VR"
  Cast To Single42/1 -> Bus Creator4/2  "L1_C1"
  Cast To Single43/1 -> Bus Creator4/1  "L1_C0"
  Cast To Single59/1 -> Bus Creator4/7  "L1_Type"
  Cast To Single58/1 -> Subsystem1/1(L1_Q_In)  "L1_Q"
  Cast To Single44/1 -> Bus Creator4/3  "L1_C2"
  Cast To Single75/1 -> Bus Creator3/8  "R0_W"
  Cast To Single60/1 -> Bus Creator3/4  "R0_C3"
  Cast To Single57/1 -> Bus Creator3/5  "R0_VR"
  Cast To Single48/1 -> Bus Creator3/7  "R0_Type"
  Cast To Single47/1 -> Subsystem/1(R0_Q_In)  "R0_Q"
  Cast To Single55/1 -> Bus Creator3/1  "R0_C0"
  Cast To Single54/1 -> Bus Creator3/2  "R0_C1"
  Cast To Single56/1 -> Bus Creator3/3  "R0_C2"
  Cast To Single77/1 -> Bus Creator2/7  "L0_Type"
  Cast To Single76/1 -> Subsystem4/1(L0_Q_In)  "L0_Q"
  Cast To Single64/1 -> Bus Creator2/1  "L0_C0"
  Cast To Single65/1 -> Bus Creator2/3  "L0_C2"
  Cast To Single67/1 -> Bus Creator2/4  "L0_C3"
  Cast To Single66/1 -> Bus Creator2/5  "L0_VR"
  Cast To Single61/1 -> Bus Creator2/2  "L0_C1"
  Bus Creator2/1 -> bsL0Info/1  "bsL0Info"
  Bus Creator3/1 -> bsR0Info/1  "bsR0Info"
  Bus Creator4/1 -> bsL1Info/1  "bsL1Info"
  Bus Selector4/5 -> Cast To Single78/1  "<L1_VR>"
  Bus Selector4/2 -> Unary Minus9/1  "<L1_C1>"
  Bus Selector3/5 -> Cast To Single57/1  "<R0_VR>"
  Subsystem4/1(L0_Q) -> Bus Creator2/6
  Bus Selector4/1 -> Unary Minus8/1  "<L1_C0>"
  Bus Selector2/4 -> Unary Minus3/1  "<L0_C3>"
  Bus Selector2/6 -> Cast To Single76/1  "<L0_Q>"
  bsFusR1Info/1 -> Bus Selector5/1
  bsFusL1Info/1 -> Bus Selector4/1
  bsFusR0Info/1 -> Bus Selector3/1
  Bus Selector4/7 -> Cast To Single59/1  "<L1_Type>"
  bsFusL0Info/1 -> Bus Selector2/1
  Bus Selector2/3 -> Unary Minus2/1  "<L0_C2>"
  Bus Selector5/1 -> Unary Minus14/1  "<R1_C0>"
  Bus Selector3/8 -> Cast To Single75/1  "<R0_W>"
  Bus Selector3/7 -> Cast To Single48/1  "<R0_Type>"
  Bus Selector3/3 -> Unary Minus6/1  "<R0_C2>"
  Bus Selector5/7 -> Cast To Single70/1  "<R1_Type>"
  Bus Selector5/6 -> Cast To Single69/1  "<R1_Q>"
  Bus Selector5/5 -> Cast To Single50/1  "<R1_VR>"
  Bus Selector2/5 -> Cast To Single66/1  "<L0_VR>"
  Bus Selector2/1 -> Unary Minus/1  "<L0_C0>"
  Bus Selector3/4 -> Unary Minus7/1  "<R0_C3>"
  Bus Selector2/8 -> Cast To Single71/1  "<L0_W>"
  Bus Selector3/2 -> Unary Minus5/1  "<R0_C1>"
  Bus Selector3/1 -> Unary Minus4/1  "<R0_C0>"
  Bus Selector2/2 -> Unary Minus1/1  "<L0_C1>"
  Bus Selector4/4 -> Unary Minus11/1  "<L1_C3>"
  Bus Selector4/6 -> Cast To Single58/1  "<L1_Q>"
  Bus Selector2/7 -> Cast To Single77/1  "<L0_Type>"
  Subsystem/1(R0_Q) -> Bus Creator3/6
  Bus Selector3/6 -> Cast To Single47/1  "<R0_Q>"
  Bus Selector5/4 -> Unary Minus13/1  "<R1_C3>"
  Bus Creator5/1 -> bsR1Info/1  "bsR1Info"
  Bus Selector5/8 -> Cast To Single52/1  "<R1_W>"
  Bus Selector5/2 -> Unary Minus15/1  "<R1_C1>"
  Bus Selector5/3 -> Unary Minus12/1  "<R1_C2>"
  Bus Selector4/8 -> Cast To Single74/1  "<L1_W>"
  Bus Selector4/3 -> Unary Minus10/1  "<L1_C2>"

== system LKAS_AutoSave_DF_20220408_1006_SW62/LKAS/LL/LL Inputs Mapping/bsLaneInfo/LanesReconstruct  ==
  bsLLClb : Inport
  bsL0Info : Inport  Port=2
  bsR0Info : Inport  Port=3
  bsL1Info : Inport  Port=4
  bsR1Info : Inport  Port=5
  bsLrgInfo : Inport  Port=6
  bsRrgInfo : Inport  Port=7
  Bus Selector5 : BusSelector  OutputSignals=L0_Q
  Bus Selector6 : BusSelector  OutputSignals=R0_Q
  LaneReconstructSM : Stateflow chart  TreatAsAtomicUnit=on
  Left 1Lane Reconstruct (Lft1LaneR) : Subsystem
  Left Lane Reconstruct (LftLaneR) : Subsystem
  Right 1Lane Reconstruct (Rgt1LaneR) : Subsystem
  Right Lane Reconstruct (RgtLaneR) : Subsystem
  RoadSide Offset : Subsystem
  Switch : Switch  Criteria=u2 > Threshold
  Switch1 : Switch  Criteria=u2 > Threshold
  bsL0InfoR : Outport
  bsR0InfoR : Outport  Port=2
  bsL1InfoR : Outport  Port=3
  bsR1InfoR : Outport  Port=4
  wires:
  bsRrgInfo/1 -> RoadSide Offset/4(bsRrgInfo)
  bsLrgInfo/1 -> RoadSide Offset/3(bsLrgInfo)
  bsLLClb/1 -> RoadSide Offset/5(bsLLClb)
  RoadSide Offset/2(bsR0Infoout) -> Bus Selector6/1, Left Lane Reconstruct (LftLaneR)/2(bsR0Info), Right Lane Reconstruct (RgtLaneR)/2(bsR0Info), Switch/1
  RoadSide Offset/1(bsL0Infoout) -> Bus Selector5/1, Right Lane Reconstruct (RgtLaneR)/1(bsL0Info), Switch1/1, Left Lane Reconstruct (LftLaneR)/3(bsL0Info)
  bsL0Info/1 -> RoadSide Offset/1(bsL0Info)
  bsR0Info/1 -> RoadSide Offset/2(bsR0Info)
  [LftFlg] -> Switch1/2
  [RgtFlg] -> Switch/2
  [LftFlg] -> Left 1Lane Reconstruct (Lft1LaneR)/1(stFlag)
  [RgtFlg] -> Right 1Lane Reconstruct (Rgt1LaneR)/1(stFlag)
  Left 1Lane Reconstruct (Lft1LaneR)/1(bsL1InfoR) -> bsL1InfoR/1
  Right 1Lane Reconstruct (Rgt1LaneR)/1(bsL1InfoR) -> bsR1InfoR/1
  bsR1Info/1 -> Right 1Lane Reconstruct (Rgt1LaneR)/2(bsR1Info)
  LaneReconstructSM/3(LaneRSM_stRgtFlg) -> [RgtFlg]
  LaneReconstructSM/2(LaneRSM_stLftFlg) -> [LftFlg]
  LaneReconstructSM/1(LaneRSM_stRoadFlg) -> [RoadFlg]
  Switch1/1 -> bsL0InfoR/1
  Switch/1 -> bsR0InfoR/1
  Right Lane Reconstruct (RgtLaneR)/1(bsR0InfoR) -> Switch/3
  Left Lane Reconstruct (LftLaneR)/1(bsL0InfoR) -> Switch1/3
  RoadSide Offset/3(lRoadW) -> [RoadWidth], Right Lane Reconstruct (RgtLaneR)/3(lRoadW), Left Lane Reconstruct (LftLaneR)/1(lRoadW)
  Bus Selector5/1 -> LaneReconstructSM/1(LaneRSM_stL0Ql)  "<L0_Q>"
  Bus Selector6/1 -> LaneReconstructSM/2(LaneRSM_stR0Ql)  "<R0_Q>"
  bsL1Info/1 -> Left 1Lane Reconstruct (Lft1LaneR)/2(bsL1Info)

== system LKAS_AutoSave_DF_20220408_1006_SW62/LKAS/LL/LLOn/LDW/Heading Angle Detection (HdAgDet) ==
  Enable : Inport
  phiHdAg_Lft : Inport  Port=2
  phiHdAg_Rgt : Inport  Port=3
  LL_LDWS_SUPPRESS_HEADING : Inport  Port=4
  LKA_SampleTime : Inport  Port=5
  Constant : Constant  Value=0.05  OutDataTypeStr=single
  If : If  IfExpression=u1==1  ElseIfExpressions=u1==2
  If Action Subsystem : Subsystem  TreatAsAtomicUnit=on
  If Action Subsystem1 : Subsystem  TreatAsAtomicUnit=on
  If Action Subsystem2 : Subsystem  TreatAsAtomicUnit=on
  Merge : Merge  Inputs=3  InitialOutput=0
  Relational Operator : RelationalOperator  OutDataTypeStr=boolean  RndMeth=Nearest
  Sum Condition : Subsystem
  stHdAgDetFlg : Outport
  wires:
  Sum Condition/1(Out) -> stHdAgDetFlg/1
  Constant/1 -> Sum Condition/2(Sum)
  Relational Operator/1 -> Sum Condition/Enable
  LL_LDWS_SUPPRESS_HEADING/1 -> Relational Operator/2
  Merge/1 -> Relational Operator/1
  Enable/1 -> If/1
  phiHdAg_Rgt/1 -> If Action Subsystem1/1(In1)
  phiHdAg_Lft/1 -> If Action Subsystem/1(In1)
  If/3 -> If Action Subsystem2/Action
  If Action Subsystem2/1(Out1) -> Merge/3
  If/2 -> If Action Subsystem1/Action
  If Action Subsystem1/1(Out1) -> Merge/2
  If Action Subsystem/1(Out1) -> Merge/1
  If/1 -> If Action Subsystem/Action
  LKA_SampleTime/1 -> Sum Condition/1(In)

== system LKAS_AutoSave_DF_20220408_1006_SW62/LKAS/LL/LLOn/LKA/Driver Torque Addition (DTA) ==
  DTA_bsInInfoSyn : Inport
  DTA_bsLFClb : Inport  Port=2
  DTA_Exit3Flg : Inport  Port=3
  Bus Selector : BusSelector  OutputSignals=bsLKAClb.LL_LKASWAClb.LL_LKASWASyn_TrqSwaAddSwt
  Compare To Constant : simulink/Logic and Bit Operations/Compare To Constant  relop=>  const=0  OutDataTypeStr=boolean
  Driver Torque Assist : Subsystem
  Subsystem : Subsystem
  DTA_phiDTASWACmd : Outport
  DTA_M : Outport  Port=2
  wires:
  DTA_Exit3Flg/1 -> Driver Torque Assist/3(DTA_Exit3Flg)
  Compare To Constant/1 -> Subsystem/Enable
  Bus Selector/1 -> Compare To Constant/1  "<LL_LKASWASyn_TrqSwaAddSwt>"
  Driver Torque Assist/1(DTA_M) -> DTA_M/1
  Subsystem/1(DTA_phiDTASWACmd) -> DTA_phiDTASWACmd/1
  DTA_bsLFClb/1 -> Subsystem/2(DTA_bsLFClb), Bus Selector/1, Driver Torque Assist/2(DTA_bsLFClb)
  DTA_bsInInfoSyn/1 -> Driver Torque Assist/1(DTA_bsInInfoSyn), Subsystem/1(DTA_bsInInfoSyn)
